simulink model "Dyn3DoF_dv_test"  (R2018b)
settings: configuration reference "Configuration" (kept outside this file)
model workspace (MATLAB code in the model file):
  | CON = Simulink.Parameter;
  | CON.DataType = 'Bus: Bus_CON';
  | CON.Value = Simulink.Bus.createMATLABStruct('Bus_CON');
  | 
  | sat = Simulink.Parameter;
  | sat.DataType = 'Bus: Bus_sat';
  | sat.Value = Simulink.Bus.createMATLABStruct('Bus_sat');
undefined symbols (not defined in the file): TimeStep
settings Model: ParameterArgumentNames=CON,sat  OrderedModelArguments=off  Creator=Ethan  LastModifiedBy=Ethan
settings ConfigSetRef: SourceLocation=Base Workspace

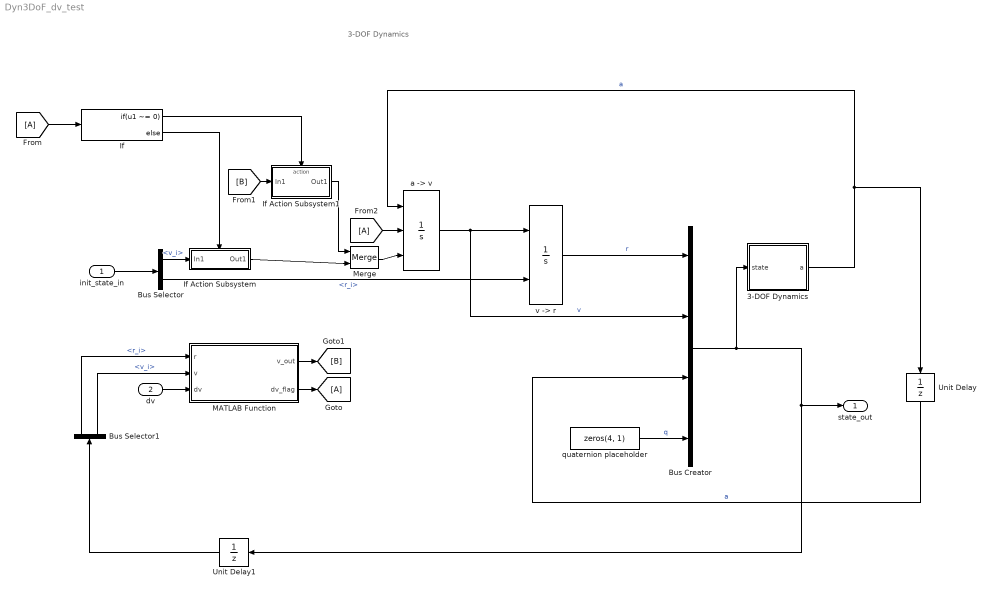
== system Dyn3DoF_dv_test ==
  note: 3-DOF Dynamics
  init_state_in : Inport  OutDataTypeStr=Bus: Bus_state
  dv : Inport  Port=2  OutDataTypeStr=double  PortDimensions=3
  3-DOF Dynamics : MATLAB Function  TreatAsAtomicUnit=on
  Bus Creator : BusCreator  Inputs=4  OutDataTypeStr=Bus: Bus_state  NonVirtualBus=on
      settings: InheritFromInputs=off
  Bus Selector : BusSelector  OutputSignals=v_i,r_i
  Bus Selector1 : BusSelector  OutputSignals=r_i,v_i
  If : If  IfExpression=u1 ~= 0
  If Action Subsystem : Subsystem  TreatAsAtomicUnit=on
  If Action Subsystem1 : Subsystem  TreatAsAtomicUnit=on
  MATLAB Function : MATLAB Function  TreatAsAtomicUnit=on  SystemSampleTime=TimeStep
  Merge : Merge
  Unit Delay : UnitDelay  InitialCondition=zeros(3, 1)  SampleTime=-1
  Unit Delay1 : UnitDelay  SampleTime=-1
  "a -> v" : Integrator  ExternalReset=level hold  InitialConditionSource=external
  quaternion placeholder : Constant  Value=zeros(4, 1)
  "v -> r" : Integrator  InitialConditionSource=external
  state_out : Outport  OutDataTypeStr=Bus: Bus_state
  wires:
  init_state_in/1 -> Bus Selector/1
  3-DOF Dynamics/1(a) -> "a -> v"/1, Unit Delay/1  "a"
  Bus Creator/1 -> Unit Delay1/1, state_out/1, 3-DOF Dynamics/1(state)
  "v -> r"/1 -> Bus Creator/1  "r"
  quaternion placeholder/1 -> Bus Creator/4  "q"
  Unit Delay/1 -> Bus Creator/3  "a"
  dv/1 -> MATLAB Function/3(dv)
  Unit Delay1/1 -> Bus Selector1/1
  Bus Selector1/1 -> MATLAB Function/1(r)  "<r_i>"
  Bus Selector/2 -> "v -> r"/2  "<r_i>"
  Bus Selector1/2 -> MATLAB Function/2(v)  "<v_i>"
  "a -> v"/1 -> Bus Creator/2, "v -> r"/1  "v"
  Bus Selector/1 -> If Action Subsystem/1(In1)  "<v_i>"
  MATLAB Function/2(dv_flag) -> [A]
  [A] -> If/1
  If/2 -> If Action Subsystem/Action
  If/1 -> If Action Subsystem1/Action
  If Action Subsystem1/1(Out1) -> Merge/1
  If Action Subsystem/1(Out1) -> Merge/2
  MATLAB Function/1(v_out) -> [B]
  [B] -> If Action Subsystem1/1(In1)
  [A] -> "a -> v"/2
  Merge/1 -> "a -> v"/3

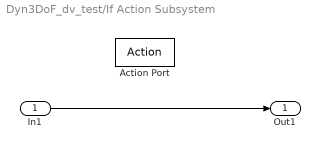
== system Dyn3DoF_dv_test/If Action Subsystem ==
  In1 : Inport
  Action Port : ActionPort  ActionType=else
  Out1 : Outport
  wires:
  In1/1 -> Out1/1

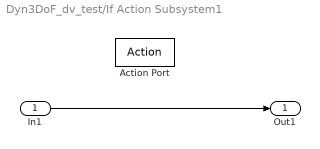
== system Dyn3DoF_dv_test/If Action Subsystem1 ==
  In1 : Inport
  Action Port : ActionPort  ActionType=then
  Out1 : Outport
  wires:
  In1/1 -> Out1/1

== matlab function Dyn3DoF_dv_test/MATLAB Function ==
  settings: updateMethod=DISCRETE
  data: r input; v_out output; v input; dv input; dv_flag output
function [v_out, dv_flag] = fcn(r,v, dv)

% persistent dv_flag_in
% if isempty(dv_flag_in)
%     dv_flag_in = 0;
% end
dv_flag_in = 0;

if any(dv ~= zeros(3, 1))
    dv_flag_in = 1;
end

v_out = v + dv;

dv_flag = dv_flag_in;

== matlab function Dyn3DoF_dv_test/3-DOF Dynamics ==
  data: state input; a output; CON parameter; sat parameter
function a = dyn(state, CON, sat)

r = state.r_i;
v = state.v_i;

a = zeros(3, 1);

if CON.gravityFlag == 0
    a = - CON.mu * r / norm(r) ^ 3;
elseif CON.gravityFlag == 1
    a(1) = - CON.mu * r(1) / norm(r) ^ 3 * (1 - CON.J2 * 3/2 * ...
        (CON.Re/norm(r))^2 * (5 * r(3)^2 / norm(r)^2 - 1));
    a(2) = - CON.mu * r(2) / norm(r) ^ 3 * (1 - CON.J2 * 3/2 * ...
        (CON.Re/norm(r))^2 * (5 * r(3)^2 / norm(r)^2 - 1));
    a(3) = - CON.mu * r(3) / norm(r) ^ 3 * (1 - CON.J2 * 3/2 * ...
        (CON.Re/norm(r))^2 * (5 * r(3)^2 / norm(r)^2 - 3));
else
    a = - CON.mu * r / norm(r) ^ 3;
end

if CON.dragFlag
    a_drag = drag_func(r, v, sat, CON);
    a = a + a_drag;
end
% i2lvlh = rv2RTN(r, v);
% a = a + i2lvlh' * dv / CON.dt;
end
